simulink model "PR9"  (R2015b)
settings: Solver=VariableStepAuto  StartTime=0.0  StopTime=200  RelTol=1e-3
libraries: simulink x1
settings Model: Creator=Zachary  LastModifiedBy=zap

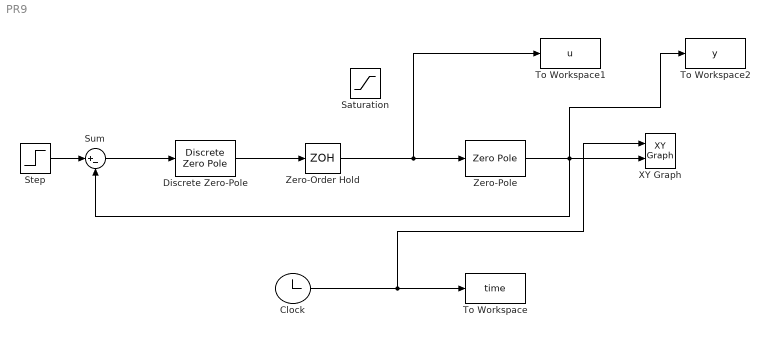
== system PR9 ==
  Clock : Clock
  Discrete Zero-Pole : DiscreteZeroPole  Zeros=[]  Poles=[]  Gain=8.1  SampleTime=0.1
  Saturation : Saturate  UpperLimit=10  LowerLimit=-10
  Step : Step  SampleTime=0.1
  Sum : Sum  Inputs=|+-
  To Workspace : ToWorkspace  VariableName=time  SaveFormat=Timeseries  SampleTime=-1
  To Workspace1 : ToWorkspace  VariableName=u  SaveFormat=Timeseries  SampleTime=-1
  To Workspace2 : ToWorkspace  VariableName=y  SaveFormat=Timeseries  SampleTime=-1
  XY Graph : simulink/Sinks/XY Graph  xmin=0  xmax=200  ymin=-5  ymax=5  st=-1
  Zero-Order Hold : ZeroOrderHold  SampleTime=0.1
  Zero-Pole : ZeroPole  Zeros=[]  Poles=[0 -0.4]
  wires:
  Discrete Zero-Pole/1 -> Zero-Order Hold/1
  Zero-Pole/1 -> Sum/2, To Workspace2/1, XY Graph/2
  Clock/1 -> To Workspace/1, XY Graph/1
  Sum/1 -> Discrete Zero-Pole/1
  Step/1 -> Sum/1
  Zero-Order Hold/1 -> To Workspace1/1, Zero-Pole/1
